simulink model "DahlinovPI"  (R2020b)
settings: Solver=VariableStepAuto  StartTime=0.0  StopTime=50  RelTol=1e-3
values from neighbouring files (symbols this model uses):
  K = 0.0829    [Parameters.m]
  Kp = (1-exp(-T/Ts))/[K0*(exp(T/T0) - 1)*(1 + N*(1 - exp(-T/Ts)))]    [Parameters.m]
settings Model: Creator=User  LastModifiedBy=user
settings DataIOCC: ReturnWorkspaceOutputs=off
settings OptimizationCC: LifeSpan=inf
settings DebuggingCC: ArithmeticOperatorsInVariantConditions=warning
settings SFSimCC: SimUseLocalCustomCode=off  CustomCodeUndefinedFunction=UseInterfaceOnly
settings RTWCC: RTWUseLocalCustomCode=off
settings CodeAppCC: StateflowObjectComments=on

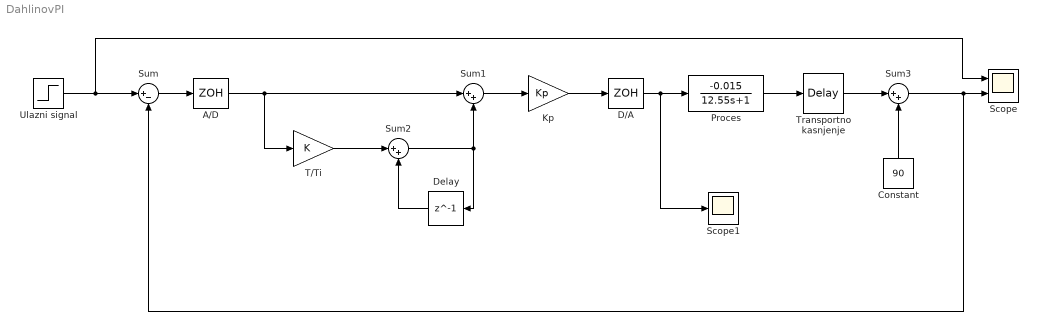
== system DahlinovPI ==
  "A/D " : ZeroOrderHold
  Constant : Constant  Value=90
  D/A : ZeroOrderHold
  Delay : Delay  DelayLength=1
  Kp : Gain  Gain=Kp
  Proces : TransferFcn  Numerator=[-0.015]  Denominator=[12.55 1]
  Scope : Scope  NumInputPorts=2
  Scope1 : Scope
  Sum : Sum  Inputs=|+-
  Sum1 : Sum  Inputs=|++
  Sum2 : Sum  Inputs=|++
  Sum3 : Sum  Inputs=|++
  T/Ti : Gain  Gain=K
  Transportno kasnjenje : TransportDelay  DelayTime=2.35
  Ulazni signal : Step  Time=5  Before=90  After=85  SampleTime=0
  wires:
  Ulazni signal/1 -> Scope/1, Sum/1
  Sum/1 -> "A/D "/1
  "A/D "/1 -> T/Ti/1, Sum1/1
  T/Ti/1 -> Sum2/1
  Sum2/1 -> Delay/1, Sum1/2
  Delay/1 -> Sum2/2
  Sum1/1 -> Kp/1
  Kp/1 -> D/A/1
  Proces/1 -> Transportno kasnjenje/1
  Transportno kasnjenje/1 -> Sum3/1
  Constant/1 -> Sum3/2
  Sum3/1 -> Scope/2, Sum/2
  D/A/1 -> Scope1/1, Proces/1
